simulink model "projekt1_8_v3"  (R2016b)
settings: Solver=VariableStepAuto  StartTime=0.0  StopTime=10.0  RelTol=1e-3
values from neighbouring files (symbols this model uses):
  A3 = a1 + 2*a2*u3_ + 3*a3*u3_^2 + 4*a4*u3_^3    (= 0.288125)    [projekt1_5.m]
  B3 = (a1*u3_ + a2*u3_^2 + a3*u3_^3 + a4*u3_^4) - A3*u3_    (= -0.03515625)    [projekt1_5.m]
  K = 3.5    [projekt1.m]    (also in projekt1_5.m)
  T1 = 4    [projekt1.m]    (also in projekt1_5.m)
  T2 = 8    [projekt1.m]    (also in projekt1_5.m)
  Tp = 1    [projekt1.m]    (also in projekt1_5.m)
settings Model: Creator=m  LastModifiedBy=m

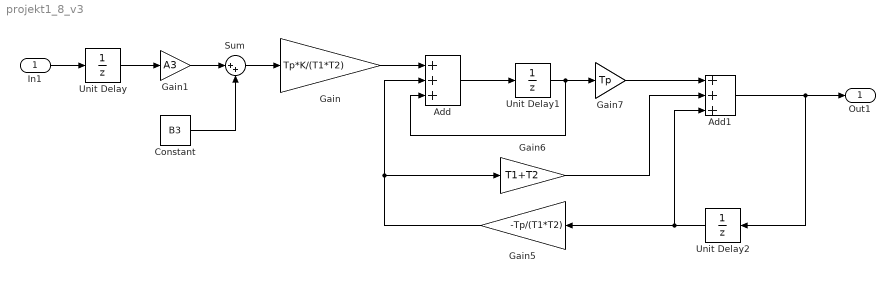
== system projekt1_8_v3 ==
  In1 : Inport
  Add : Sum  Inputs=+++
  Add1 : Sum  Inputs=+++
  Constant : Constant  Value=B3
  Gain : Gain  Gain=Tp*K/(T1*T2)
  Gain1 : Gain  Gain=A3
  Gain5 : Gain  Gain=-Tp/(T1*T2)
  Gain6 : Gain  Gain=T1+T2
  Gain7 : Gain  Gain=Tp
  Sum : Sum  Inputs=|++
  Unit Delay : UnitDelay  SampleTime=-1
  Unit Delay1 : UnitDelay  SampleTime=-1
  Unit Delay2 : UnitDelay  SampleTime=-1
  Out1 : Outport  SignalName=yl(k)
  wires:
  Gain/1 -> Add/1
  Gain5/1 -> Add/2, Gain6/1
  In1/1 -> Unit Delay/1
  Add/1 -> Unit Delay1/1
  Unit Delay1/1 -> Add/3, Gain7/1
  Gain6/1 -> Add1/2
  Gain7/1 -> Add1/1
  Add1/1 -> Unit Delay2/1, Out1/1
  Unit Delay2/1 -> Add1/3, Gain5/1
  Sum/1 -> Gain/1
  Gain1/1 -> Sum/1
  Unit Delay/1 -> Gain1/1
  Constant/1 -> Sum/2
